simulink model "sim_pla"  (Simulink 2.20)
settings: Solver=FixedStepDiscrete  StartTime=0.0  StopTime=200  MaxStep=.1  RelTol=1e-5  AbsTol=1e-5
values from neighbouring files (symbols this model uses):
  Btot_p = [1.01219559056 -0.470264843111 0.0164957191282 0.00637641130362 -0.0114044125868 0.0367191858533 0.00475496453764 0.0142682114975 -0.02612243686 0.00492786107634 -0.0232059691443 0.00221978390651 ... (36 elements, 6x6)]    [Plant_da.mat]
  Btot_s = [-1.01626574689 2.87547182252 0.160783159509 -0.0616056082235 0.415835595232 -0.0519110171366 -0.981144722525 0.331237826324 0.0458866161445 0.0273695758621 -0.450541570766 0.161910461736 ... (36 elements, 6x6)]    [Plant_da.mat]
  Dtot_p = [0.513358369793  0.0351099859011  0.00780615785705; 0.00923678162985  0.40412781442  0.00373697732041; 0.000710321631108  0.27377444097  0.302765835746]    [Plant_da.mat]
  Dtot_s = [1.88799295885 1.15607702775 1.0967215675 -0.0862589557053 -0.000817934293654 -0.111851597277 2.17273827487 1.17822487272 1.10291377498 0.0376770859254 -0.0289504261378 0.0426395979727 ... (18 elements, 3x6)]    [Plant_da.mat]
  Ftot_p = [-10 5 0 0 0 0 -5 2.40692882292e-15 0 0 0 0 ... (36 elements, 6x6)]    [Plant_da.mat]
  Ftot_s = [-20 10 0 0 0 0 -10 5.05150120952e-15 0 0 0 0 ... (36 elements, 6x6)]    [Plant_da.mat]
  knot_a3_p = [200 1400]    [Plant_da.mat]
  knot_a3_s = [200 1400]    [Plant_da.mat]
  knot_a5_p = [200 1400]    [Plant_da.mat]
  knot_a5_s = [0 1]    [Plant_da.mat]
  knot_d_p = [200 1400]    [Plant_da.mat]
  knot_d_s = [0 1]    [Plant_da.mat]
  knot_u_p = [200 1400]    [Plant_da.mat]
  knot_u_s = [0 1]    [Plant_da.mat]
  knot_y_p = [200 1400]    [Plant_da.mat]
  knot_y_s = [200 1400]    [Plant_da.mat]
  Ltot_p = [-1.64126952333 0.984947018254 0 0 0 0 -0.233477858246 0.0041951537679 0 0 0 0 ... (54 elements, 6x9)]    [Plant_da.mat]
  Ltot_s = [-2.86862859726 1.57424910459 0 0 0 0 -0.0579168602778 -0.011710441158 0 0 0 0 ... (72 elements, 6x12)]    [Plant_da.mat]
  M3_p = [-0.061197222075 8.55026347734 0 0 0 0 7.49858890056 23.7640569756 0 0 0 0 ... (72 elements, 6x12)]    [Plant_da.mat]
  M3_s = [-0.00930250944473 1.93496177148 0 0 0 0 -0.0214766871049 10.7782036277 0 0 0 0 ... (36 elements, 6x6)]    [Plant_da.mat]
  M5_p = [9.76740961374 0 0 -13.0234685756 0 0 -3.35875871132 0 0 0 -0.663402612193 0 ... (27 elements, 3x9)]    [Plant_da.mat]
  M5_s = [-3.17982066424  0  0; 0  -1.6903608647  0; 0  0  -1.55540118092]    [Plant_da.mat]
  ninp_p = 3    [Plant_da.mat]
  ninp_s = 3    [Plant_da.mat]
  noutp_p = 3    [Plant_da.mat]
  noutp_s = 3    [Plant_da.mat]
  order_a3_p = [0 1 2 3]    [Plant_da.mat]
  order_a3_s = [0 1]    [Plant_da.mat]
  order_a5_p = [0 1 2]    [Plant_da.mat]
  order_a5_s = 1    [Plant_da.mat]
  order_d_p = 0    [Plant_da.mat]
  order_d_s = [0 1]    [Plant_da.mat]
  order_u_p = [0 3]    [Plant_da.mat]
  order_u_s = [0 1]    [Plant_da.mat]
  order_y_p = [0 1 3]    [Plant_da.mat]
  order_y_s = [0 1 2 3]    [Plant_da.mat]
  TSAMPLEP = 0.00833333333333    [Plant_da.mat]
  xx0_p = [-43.6952648027 46.4302892278 -75.6051233614 37.0208850933 -65.9903404423 60.1627507041]    [Plant_da.mat]
  xx0_s = [-76.0618282874 11.7629910946 -77.2669838113 13.8232604668 -77.7589073013 10.6536765168]    [Plant_da.mat]
undefined symbols (not defined in the file or in its folder): legev_bv
settings Model: SaveTime=off  SaveOutput=off  ConsistencyChecking=off  RTWPlaceOutputsASAP=off

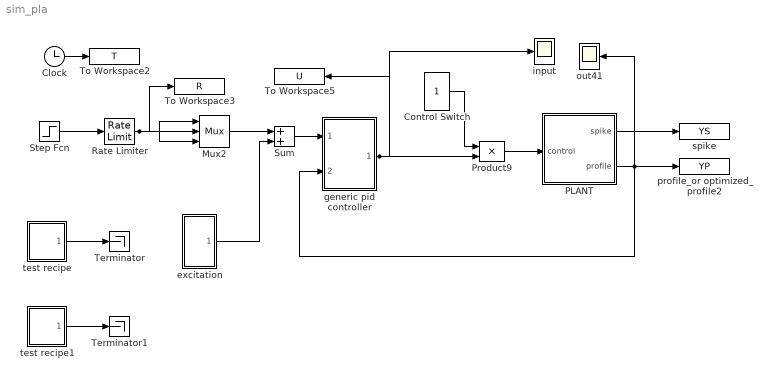
== system sim_pla ==
  Clock : Clock
  Control Switch : Constant  Value=1
  Mux2 : Mux  Inputs=3
  PLANT : Subsystem
      mask init:
      | load 'plant_da'
  Product9 : Product  Inputs=2
  Rate Limiter : RateLimiter  RisingSlewLimit=15  FallingSlewLimit=-5
  Step Fcn : Step  Time=30  Before=550  After=800
  Sum : Sum  Inputs=++
  Terminator : Terminator
  Terminator1 : Terminator
  To Workspace2 : ToWorkspace  VariableName=T  SampleTime=0
      settings: Buffer=25000
  To Workspace3 : ToWorkspace  VariableName=R  SampleTime=0
      settings: Buffer=25000
  To Workspace5 : ToWorkspace  VariableName=U  SampleTime=0
      settings: Buffer=25000
  excitation : Subsystem
      mask init:
      | load 'excit'
  generic pid controller : Subsystem
  input : Scope
      settings: TickLabels=on  TimeRange=200  YMin=0  YMax=1  SaveToWorkspace=off  SaveName=ScopeData  MaxRows=25000  SampleInput=on
  out41 : Scope
      settings: TickLabels=on  TimeRange=200  YMin=500  YMax=1000  SaveToWorkspace=off  SaveName=ScopeData  MaxRows=25000  SampleInput=on
  profile_or optimized_profile2 : ToWorkspace  VariableName=YP  SampleTime=0
      settings: Buffer=25000
  spike : ToWorkspace  VariableName=YS  SampleTime=0
      settings: Buffer=25000
  test recipe : Subsystem  mask(Repeating table){@1=[0     20    35  95  96  200], @2=[550 550 800 800 600 600]}
      mask prompts: @1 "Time values:"; @2 "Output values:"
      mask help:
      | Repeating table.
      | Enter values of time and output for first cycle.
      mask init:
      | period = max(@1); t = @1; y = @2;
      mask Help: Repeats cycle given in table. Time values should be monotonically increasing.
      mask Display: plot([t,t+period,t+2*period],[y,y,y])
  test recipe1 : Subsystem  mask(Repeating table){@1=[0     20    21  95  96  200], @2=[550 550 800 800 600 600]}
      mask prompts: @1 "Time values:"; @2 "Output values:"
      mask help:
      | Repeating table.
      | Enter values of time and output for first cycle.
      mask init:
      | period = max(@1); t = @1; y = @2;
      mask Help: Repeats cycle given in table. Time values should be monotonically increasing.
      mask Display: plot([t,t+period,t+2*period],[y,y,y])
  wires:
  Clock/1 -> To Workspace2/1
  Control Switch/1 -> Product9/1
  Product9/1 -> PLANT/1(control)
  Rate Limiter/1 -> To Workspace3/1, Mux2/1, Mux2/2, Mux2/3
  generic pid controller/1(out_1) -> Product9/2, To Workspace5/1, input/1
  Mux2/1 -> Sum/1
  Sum/1 -> generic pid controller/1(reference)
  PLANT/2(profile) -> generic pid controller/2(output), profile_or optimized_profile2/1, out41/1
  PLANT/1(spike) -> spike/1
  excitation/1(Out1) -> Sum/2
  test recipe/1(out_1) -> Terminator/1
  Step Fcn/1 -> Rate Limiter/1
  test recipe1/1(out_1) -> Terminator1/1

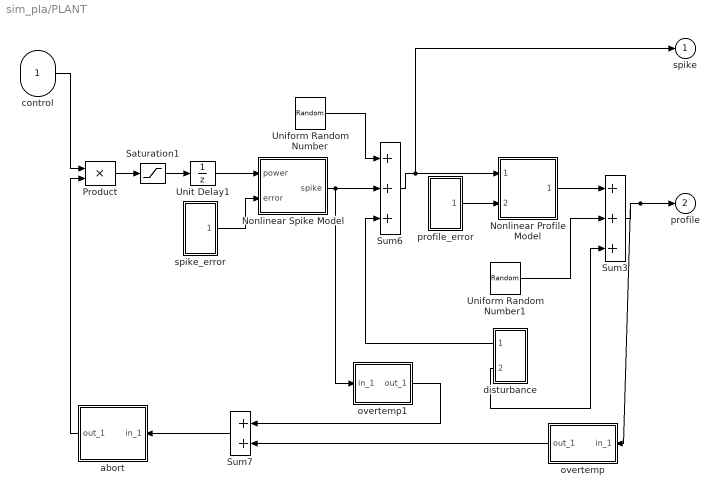
== system sim_pla/PLANT ==
  control : Inport  Port=1  PortWidth=-1  SampleTime=-1
  Nonlinear Profile Model : Subsystem
  Nonlinear Spike Model : Subsystem
  Product : Product  Inputs=2
  Saturation1 : Saturate  UpperLimit=[1 1 1]  LowerLimit=[0 0 0]
  Sum3 : Sum  Inputs=+++
  Sum6 : Sum  Inputs=+++
  Sum7 : Sum  Orientation=left  Inputs=++
  Uniform Random Number : UniformRandomNumber  Minimum=-.2  Maximum=.2  Seed=0  SampleTime=.5/60
  Uniform Random Number1 : UniformRandomNumber  Minimum=-.1  Maximum=.1  Seed=0  SampleTime=.5/60
  Unit Delay1 : UnitDelay  X0=0  SampleTime=TSAMPLEP
  abort : Subsystem  Orientation=left
  disturbance : Subsystem  Orientation=left
  overtemp : Subsystem  Orientation=left
  overtemp1 : Subsystem
  profile_error : Subsystem
  spike_error : Subsystem
  spike : Outport  Port=1  InitialOutput=0
  profile : Outport  Port=2  InitialOutput=0
  wires:
  Nonlinear Profile Model/1(profile) -> Sum3/1
  Uniform Random Number/1 -> Sum6/1
  Product/1 -> Saturation1/1
  Saturation1/1 -> Unit Delay1/1
  Unit Delay1/1 -> Nonlinear Spike Model/1(power)
  control/1 -> Product/1
  spike_error/1(out_1) -> Nonlinear Spike Model/2(error)
  profile_error/1(out_1) -> Nonlinear Profile Model/2(error)
  Uniform Random Number1/1 -> Sum3/2
  Nonlinear Spike Model/1(spike) -> Sum6/2, overtemp1/1(in_1)
  Sum3/1 -> profile/1, overtemp/1(in_1)
  Sum6/1 -> Nonlinear Profile Model/1(spike1), spike/1
  abort/1(out_1) -> Product/2
  Sum7/1 -> abort/1(in_1)
  overtemp1/1(out_1) -> Sum7/1
  overtemp/1(out_1) -> Sum7/2
  disturbance/1(spike) -> Sum6/3
  disturbance/2(profile) -> Sum3/3

== system sim_pla/excitation ==
  From  Workspace : FromWorkspace  VariableName=[TX,RX]
  Gain : Gain  Gain=1
  Out1 : Outport  Port=1  InitialOutput=0
  wires:
  Gain/1 -> Out1/1
  From  Workspace/1 -> Gain/1

== system sim_pla/generic pid controller ==
  note: 2.9873e-002  2.3770e+000  1.1004e+000
      |   5.8485e-002  3.6863e+000  1.3216e+000
      |   3.1318e-002  1.7040e+000  2.9610e+000
  reference : Inport  Port=1  PortWidth=-1  SampleTime=-1
  output : Inport  Port=2  PortWidth=-1  SampleTime=-1
  "AW-PID " : Subsystem  mask(Anti-windup PID ){SAM=.1, TF=0.1, DT=.5/60}
      mask prompts: SAM "Gain kp - Integral time ki - Derivative time kd"; TF "Pseudo-derivative filter time constant"; DT "Error lowpass filter Time constant"
      mask help: Discrete PID with Anti-windup and with lowpass filter
      mask init:
      | kp=@1(1);ki=@1(2);kd=@1(3);umax=@5(1);umin=@5(2);
      mask Display: disp('AW-PID+filter')
  AW-PID 1 : Subsystem  mask(Anti-windup PID ){@1=[.047, 1.96, 1.2], @2=.1, @3=0.1, @4=.5/60, @5=[1 0]}
      mask prompts: @1 "Gain kp - Integral time ki - Derivative time kd"; @2 "Pseudo-derivative filter time constant"; @3 "Error lowpass filter Time constant"; @4 "Sampling Time"; @5 "Saturation Limits [umax umin]"
      mask help: Discrete PID with Anti-windup and with lowpass filter
      mask init:
      | kp=@1(1);ki=@1(2);kd=@1(3);SAM=@2;TF=@3;DT=@4;umax=@5(1);umin=@5(2);
      mask Display: disp('AW-PID+filter')
  AW-PID 2 : Subsystem  mask(Anti-windup PID ){@1=[.027, 1.66, 1.9], @2=.1, @3=0.1, @4=.5/60, @5=[1 0]}
      mask prompts: @1 "Gain kp - Integral time ki - Derivative time kd"; @2 "Pseudo-derivative filter time constant"; @3 "Error lowpass filter Time constant"; @4 "Sampling Time"; @5 "Saturation Limits [umax umin]"
      mask help: Discrete PID with Anti-windup and with lowpass filter
      mask init:
      | kp=@1(1);ki=@1(2);kd=@1(3);SAM=@2;TF=@3;DT=@4;umax=@5(1);umin=@5(2);
      mask Display: disp('AW-PID+filter')
  Demux : Demux  Outputs=3
  Demux1 : Demux  Outputs=3
  Mux2 : Mux  Inputs=3
  out_1 : Outport  Port=1  InitialOutput=0
  wires:
  AW-PID 2/1(Input to system) -> Mux2/3
  "AW-PID "/1(Input to system) -> Mux2/1
  AW-PID 1/1(Input to system) -> Mux2/2
  Mux2/1 -> out_1/1
  reference/1 -> Demux/1
  Demux/1 -> "AW-PID "/1(Set point)
  Demux/2 -> AW-PID 1/1(Set point)
  Demux/3 -> AW-PID 2/1(Set point)
  Demux1/3 -> AW-PID 2/2(System Output)
  output/1 -> Demux1/1
  Demux1/2 -> AW-PID 1/2(System Output)
  Demux1/1 -> "AW-PID "/2(System Output)

== system sim_pla/test recipe ==
  Clock : Clock
  Fcn1 : Fcn  Expr=rem(u[1],period)
  Look-Up Table : Lookup  InputValues=t  OutputValues=y
  out_1 : Outport  Port=1  InitialOutput=0
  wires:
  Look-Up Table/1 -> out_1/1
  Clock/1 -> Fcn1/1
  Fcn1/1 -> Look-Up Table/1

== system sim_pla/test recipe1 ==
  Clock : Clock
  Fcn1 : Fcn  Expr=rem(u[1],period)
  Look-Up Table : Lookup  InputValues=t  OutputValues=y
  out_1 : Outport  Port=1  InitialOutput=0
  wires:
  Look-Up Table/1 -> out_1/1
  Clock/1 -> Fcn1/1
  Fcn1/1 -> Look-Up Table/1

== system sim_pla/PLANT/Nonlinear Profile Model ==
  spike1 : Inport  Port=1  PortWidth=-1  SampleTime=-1
  error : Inport  Port=2  PortWidth=-1  SampleTime=-1
  Denominator Block : Subsystem  Orientation=left
  Numerator Block : Subsystem
  Sum : Sum  Inputs=+++
  profile : Outport  Port=1  InitialOutput=0
  wires:
  Sum/1 -> profile/1, Denominator Block/1(in_1)
  Numerator Block/1(out_1) -> Sum/1
  spike1/1 -> Numerator Block/1(in_1)
  Denominator Block/1(out_1) -> Sum/3
  error/1 -> Sum/2

== system sim_pla/PLANT/Nonlinear Spike Model ==
  power : Inport  Port=1  PortWidth=-1  SampleTime=-1
  error : Inport  Port=2  PortWidth=-1  SampleTime=-1
  Denominator Block : Subsystem  Orientation=left
  Numerator Block : Subsystem
  Sum : Sum  Inputs=+++
  spike : Outport  Port=1  InitialOutput=0
  wires:
  power/1 -> Numerator Block/1(in_1)
  Numerator Block/1(out_1) -> Sum/1
  Sum/1 -> spike/1, Denominator Block/1(in_1)
  Denominator Block/1(out_1) -> Sum/3
  error/1 -> Sum/2

== system sim_pla/PLANT/abort ==
  in_1 : Inport  Port=1  PortWidth=-1  SampleTime=-1
  Abs : Abs
  Constant : Constant  Value=1
  Relational Operator : RelationalOperator  Operator=>=
  Sum : Sum  Inputs=++
  Sum1 : Sum  Inputs=-+
  Unit Delay3 : UnitDelay  X0=0  SampleTime=TSAMPLEP
  out_1 : Outport  Port=1  InitialOutput=0
  wires:
  Sum1/1 -> out_1/1
  Relational Operator/1 -> Sum1/1
  Constant/1 -> Sum1/2, Relational Operator/2
  Unit Delay3/1 -> Relational Operator/1, Sum/2
  in_1/1 -> Abs/1
  Sum/1 -> Unit Delay3/1
  Abs/1 -> Sum/1

== system sim_pla/PLANT/disturbance ==
  Discrete Transfer Fcn : DiscreteTransferFcn  Orientation=left  Numerator=[1]  Denominator=[.5/TSAMPLEP 1-.5/TSAMPLEP]  SampleTime=TSAMPLEP
  Discrete Transfer Fcn1 : DiscreteTransferFcn  Orientation=left  Numerator=[10/TSAMPLEP -10/TSAMPLEP]  Denominator=[10/TSAMPLEP 1-10/TSAMPLEP]  SampleTime=TSAMPLEP
  Discrete Transfer Fcn2 : DiscreteTransferFcn  Orientation=left  Numerator=[1]  Denominator=[2/TSAMPLEP 1-2/TSAMPLEP]  SampleTime=TSAMPLEP
  Sum4 : Sum  Orientation=left  Inputs=++
  disturbance : Step  Orientation=left  Time=55  Before=0  After=10
  disturbance2 : Step  Orientation=left  Time=75  Before=0  After=-5
  spike : Outport  Orientation=left  Port=1  InitialOutput=0
  profile : Outport  Orientation=left  Port=2  InitialOutput=0
  wires:
  Discrete Transfer Fcn1/1 -> profile/1
  Discrete Transfer Fcn/1 -> spike/1
  Sum4/1 -> Discrete Transfer Fcn/1, Discrete Transfer Fcn1/1
  disturbance/1 -> Sum4/1
  disturbance2/1 -> Discrete Transfer Fcn2/1
  Discrete Transfer Fcn2/1 -> Sum4/2

== system sim_pla/PLANT/overtemp ==
  in_1 : Inport  Port=1  PortWidth=-1  SampleTime=-1
  Constant : Constant  Value=950
  Relational Operator : RelationalOperator  Operator=>
  out_1 : Outport  Port=1  InitialOutput=0
  wires:
  in_1/1 -> Relational Operator/1
  Relational Operator/1 -> out_1/1
  Constant/1 -> Relational Operator/2

== system sim_pla/PLANT/overtemp1 ==
  in_1 : Inport  Port=1  PortWidth=-1  SampleTime=-1
  Constant : Constant  Value=1000
  Relational Operator : RelationalOperator  Operator=>
  out_1 : Outport  Port=1  InitialOutput=0
  wires:
  in_1/1 -> Relational Operator/1
  Relational Operator/1 -> out_1/1
  Constant/1 -> Relational Operator/2

== system sim_pla/PLANT/profile_error ==
  Mux1 : Mux  Inputs=3
  prof error : Subsystem  mask(Repeating table){@1=TEPRO, @2=FEP1}
      mask prompts: @1 "Time values:"; @2 "Output values:"
      mask help:
      | Repeating table.
      | Enter values of time and output for first cycle.
      mask init:
      | period = max(@1); t = @1; y = @2;
      mask Help: Repeats cycle given in table. Time values should be monotonically increasing.
      mask Display: plot([t,t+period,t+2*period],[y,y,y])
  prof error1 : Subsystem  mask(Repeating table){@1=TEPRO, @2=FEP2}
      mask prompts: @1 "Time values:"; @2 "Output values:"
      mask help:
      | Repeating table.
      | Enter values of time and output for first cycle.
      mask init:
      | period = max(@1); t = @1; y = @2;
      mask Help: Repeats cycle given in table. Time values should be monotonically increasing.
      mask Display: plot([t,t+period,t+2*period],[y,y,y])
  prof error2 : Subsystem  mask(Repeating table){@1=TEPRO, @2=FEP3}
      mask prompts: @1 "Time values:"; @2 "Output values:"
      mask help:
      | Repeating table.
      | Enter values of time and output for first cycle.
      mask init:
      | period = max(@1); t = @1; y = @2;
      mask Help: Repeats cycle given in table. Time values should be monotonically increasing.
      mask Display: plot([t,t+period,t+2*period],[y,y,y])
  out_1 : Outport  Port=1  InitialOutput=0
  wires:
  Mux1/1 -> out_1/1
  prof error/1(out_1) -> Mux1/1
  prof error1/1(out_1) -> Mux1/2
  prof error2/1(out_1) -> Mux1/3

== system sim_pla/PLANT/spike_error ==
  Mux1 : Mux  Inputs=3
  spike error : Subsystem  mask(Repeating table){@1=TEPRO, @2=FES1}
      mask prompts: @1 "Time values:"; @2 "Output values:"
      mask help:
      | Repeating table.
      | Enter values of time and output for first cycle.
      mask init:
      | period = max(@1); t = @1; y = @2;
      mask Help: Repeats cycle given in table. Time values should be monotonically increasing.
      mask Display: plot([t,t+period,t+2*period],[y,y,y])
  spike error1 : Subsystem  mask(Repeating table){@1=TEPRO, @2=FES2}
      mask prompts: @1 "Time values:"; @2 "Output values:"
      mask help:
      | Repeating table.
      | Enter values of time and output for first cycle.
      mask init:
      | period = max(@1); t = @1; y = @2;
      mask Help: Repeats cycle given in table. Time values should be monotonically increasing.
      mask Display: plot([t,t+period,t+2*period],[y,y,y])
  spike error2 : Subsystem  mask(Repeating table){@1=TEPRO, @2=FES3}
      mask prompts: @1 "Time values:"; @2 "Output values:"
      mask help:
      | Repeating table.
      | Enter values of time and output for first cycle.
      mask init:
      | period = max(@1); t = @1; y = @2;
      mask Help: Repeats cycle given in table. Time values should be monotonically increasing.
      mask Display: plot([t,t+period,t+2*period],[y,y,y])
  out_1 : Outport  Port=1  InitialOutput=0
  wires:
  Mux1/1 -> out_1/1
  spike error/1(out_1) -> Mux1/1
  spike error1/1(out_1) -> Mux1/2
  spike error2/1(out_1) -> Mux1/3

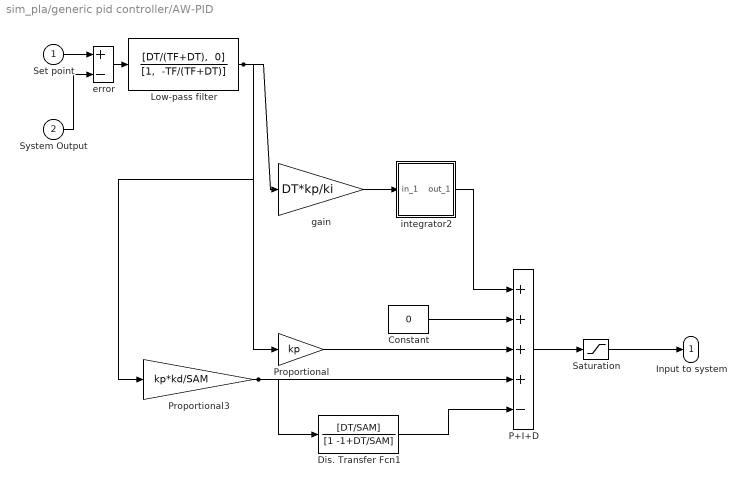
== system sim_pla/generic pid controller/AW-PID  ==
  Set point : Inport  Port=1  PortWidth=-1  SampleTime=-1
  System Output : Inport  Port=2  PortWidth=-1  SampleTime=-1
  Constant : Constant  Value=0
  Dis. Transfer Fcn1 : DiscreteTransferFcn  Numerator=[DT/SAM]  Denominator=[1 -1+DT/SAM]  SampleTime=DT
  Low-pass filter : DiscreteTransferFcn  Numerator="[DT/(TF+DT),  0]"  Denominator="[1,  -TF/(TF+DT)]"  SampleTime=DT
  P+I+D : Sum  Inputs=++++-
  Proportional : Gain  Gain=kp
  Proportional3 : Gain  Gain=kp*kd/SAM
  Saturation : Saturate  UpperLimit=umax  LowerLimit=umin
  error : Sum  Inputs=+-
  gain : Gain  Gain=DT*kp/ki
  integrator2 : Subsystem  mask(Anti windup intgrator){@1=umax, @2=umin, @3=DT}
      mask prompts: @1 "umax"; @2 "umin"; @3 "sampling time"
      mask help: Integral with anti-windup
      mask init:
      | umax=@1 ; umin =@2 ;DT=@3;
      mask Display: disp('DT-I-AW')
  Input to system : Outport  Port=1  InitialOutput=0
  wires:
  integrator2/1(out_1) -> P+I+D/1
  error/1 -> Low-pass filter/1
  Set point/1 -> error/1
  System Output/1 -> error/2
  Low-pass filter/1 -> Proportional/1, Proportional3/1, gain/1
  Dis. Transfer Fcn1/1 -> P+I+D/5
  Proportional3/1 -> Dis. Transfer Fcn1/1, P+I+D/4
  Proportional/1 -> P+I+D/3
  gain/1 -> integrator2/1(in_1)
  P+I+D/1 -> Saturation/1
  Saturation/1 -> Input to system/1
  Constant/1 -> P+I+D/2

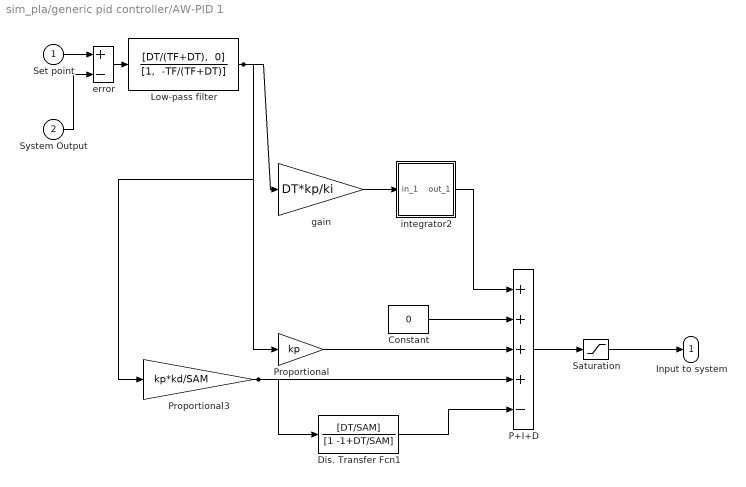
== system sim_pla/generic pid controller/AW-PID 1 ==
  Set point : Inport  Port=1  PortWidth=-1  SampleTime=-1
  System Output : Inport  Port=2  PortWidth=-1  SampleTime=-1
  Constant : Constant  Value=0
  Dis. Transfer Fcn1 : DiscreteTransferFcn  Numerator=[DT/SAM]  Denominator=[1 -1+DT/SAM]  SampleTime=DT
  Low-pass filter : DiscreteTransferFcn  Numerator="[DT/(TF+DT),  0]"  Denominator="[1,  -TF/(TF+DT)]"  SampleTime=DT
  P+I+D : Sum  Inputs=++++-
  Proportional : Gain  Gain=kp
  Proportional3 : Gain  Gain=kp*kd/SAM
  Saturation : Saturate  UpperLimit=umax  LowerLimit=umin
  error : Sum  Inputs=+-
  gain : Gain  Gain=DT*kp/ki
  integrator2 : Subsystem  mask(Anti windup intgrator){@1=umax, @2=umin, @3=DT}
      mask prompts: @1 "umax"; @2 "umin"; @3 "sampling time"
      mask help: Integral with anti-windup
      mask init:
      | umax=@1 ; umin =@2 ;DT=@3;
      mask Display: disp('DT-I-AW')
  Input to system : Outport  Port=1  InitialOutput=0
  wires:
  integrator2/1(out_1) -> P+I+D/1
  error/1 -> Low-pass filter/1
  Set point/1 -> error/1
  System Output/1 -> error/2
  Low-pass filter/1 -> Proportional/1, Proportional3/1, gain/1
  Dis. Transfer Fcn1/1 -> P+I+D/5
  Proportional3/1 -> Dis. Transfer Fcn1/1, P+I+D/4
  Proportional/1 -> P+I+D/3
  gain/1 -> integrator2/1(in_1)
  P+I+D/1 -> Saturation/1
  Saturation/1 -> Input to system/1
  Constant/1 -> P+I+D/2

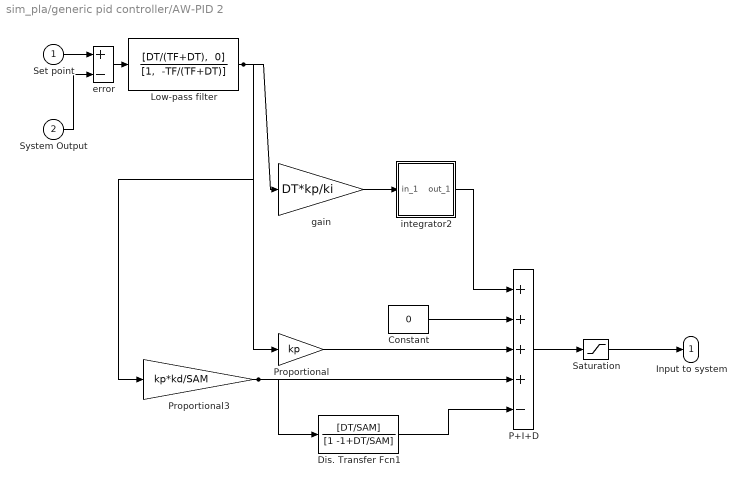
== system sim_pla/generic pid controller/AW-PID 2 ==
  Set point : Inport  Port=1  PortWidth=-1  SampleTime=-1
  System Output : Inport  Port=2  PortWidth=-1  SampleTime=-1
  Constant : Constant  Value=0
  Dis. Transfer Fcn1 : DiscreteTransferFcn  Numerator=[DT/SAM]  Denominator=[1 -1+DT/SAM]  SampleTime=DT
  Low-pass filter : DiscreteTransferFcn  Numerator="[DT/(TF+DT),  0]"  Denominator="[1,  -TF/(TF+DT)]"  SampleTime=DT
  P+I+D : Sum  Inputs=++++-
  Proportional : Gain  Gain=kp
  Proportional3 : Gain  Gain=kp*kd/SAM
  Saturation : Saturate  UpperLimit=umax  LowerLimit=umin
  error : Sum  Inputs=+-
  gain : Gain  Gain=DT*kp/ki
  integrator2 : Subsystem  mask(Anti windup intgrator){@1=umax, @2=umin, @3=DT}
      mask prompts: @1 "umax"; @2 "umin"; @3 "sampling time"
      mask help: Integral with anti-windup
      mask init:
      | umax=@1 ; umin =@2 ;DT=@3;
      mask Display: disp('DT-I-AW')
  Input to system : Outport  Port=1  InitialOutput=0
  wires:
  integrator2/1(out_1) -> P+I+D/1
  error/1 -> Low-pass filter/1
  Set point/1 -> error/1
  System Output/1 -> error/2
  Low-pass filter/1 -> Proportional/1, Proportional3/1, gain/1
  Dis. Transfer Fcn1/1 -> P+I+D/5
  Proportional3/1 -> Dis. Transfer Fcn1/1, P+I+D/4
  Proportional/1 -> P+I+D/3
  gain/1 -> integrator2/1(in_1)
  P+I+D/1 -> Saturation/1
  Saturation/1 -> Input to system/1
  Constant/1 -> P+I+D/2

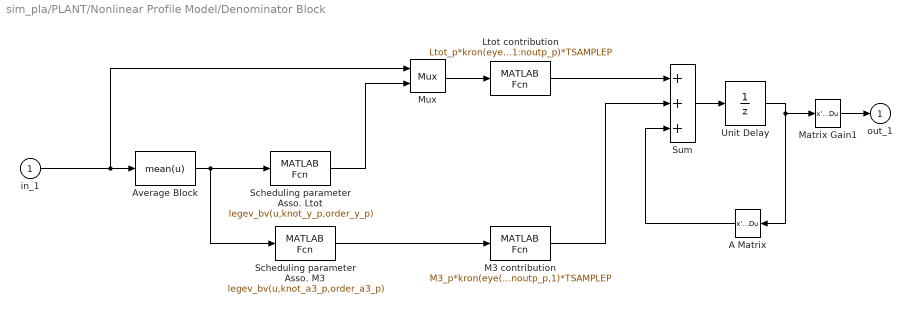
== system sim_pla/PLANT/Nonlinear Profile Model/Denominator Block ==
  in_1 : Inport  Port=1  PortWidth=-1  SampleTime=-1
  A Matrix : StateSpace  Orientation=left  A=[]  B=[]  C=[]  D=K  X0=0  mask(Matrix Gain){@1=(eye(size(Ftot_p))+TSAMPLEP*Ftot_p)}
      mask prompts: @1 "Gain matrix:"
      mask help: Matrix Gain.
      mask init:
      | K = @1;
      mask Help: Multiplies input vector by entered matrix to produce output vector (y=Au).
      mask Display: disp('K')
  Average Block : MATLABFcn  MATLABFcn=mean(u)  OutputWidth=1
  Ltot contribution : MATLABFcn  MATLABFcn=Ltot_p*kron(eye(noutp_p),u(noutp_p+1:noutp_p+length(order_y_p)))*u(1:noutp_p)*TSAMPLEP  OutputWidth=length(Ftot_p)
  M3 contribution : MATLABFcn  MATLABFcn=M3_p*kron(eye(noutp_p),u)*ones(noutp_p,1)*TSAMPLEP  OutputWidth=length(Ftot_p)
  Matrix Gain1 : StateSpace  A=[]  B=[]  C=[]  D=K  X0=0  mask(Matrix Gain){@1=Qtot_p}
      mask prompts: @1 "Gain matrix:"
      mask help: Matrix Gain.
      mask init:
      | K = @1;
      mask Help: Multiplies input vector by entered matrix to produce output vector (y=Au).
      mask Display: disp('K')
  Mux : Mux  Inputs=2
  Scheduling parameter Asso. Ltot : MATLABFcn  MATLABFcn=legev_bv(u,knot_y_p,order_y_p)  OutputWidth=length(order_y_p)
  Scheduling parameter Asso. M3 : MATLABFcn  MATLABFcn=legev_bv(u,knot_a3_p,order_a3_p)  OutputWidth=length(order_a3_p)
  Sum : Sum  Inputs=+++
  Unit Delay : UnitDelay  X0=0  SampleTime=TSAMPLEP
  out_1 : Outport  Port=1  InitialOutput=0
  wires:
  in_1/1 -> Average Block/1, Mux/1
  Average Block/1 -> Scheduling parameter Asso. Ltot/1, Scheduling parameter Asso. M3/1
  Unit Delay/1 -> A Matrix/1, Matrix Gain1/1
  A Matrix/1 -> Sum/3
  Scheduling parameter Asso. M3/1 -> M3 contribution/1
  M3 contribution/1 -> Sum/2
  Ltot contribution/1 -> Sum/1
  Scheduling parameter Asso. Ltot/1 -> Mux/2
  Mux/1 -> Ltot contribution/1
  Sum/1 -> Unit Delay/1
  Matrix Gain1/1 -> out_1/1

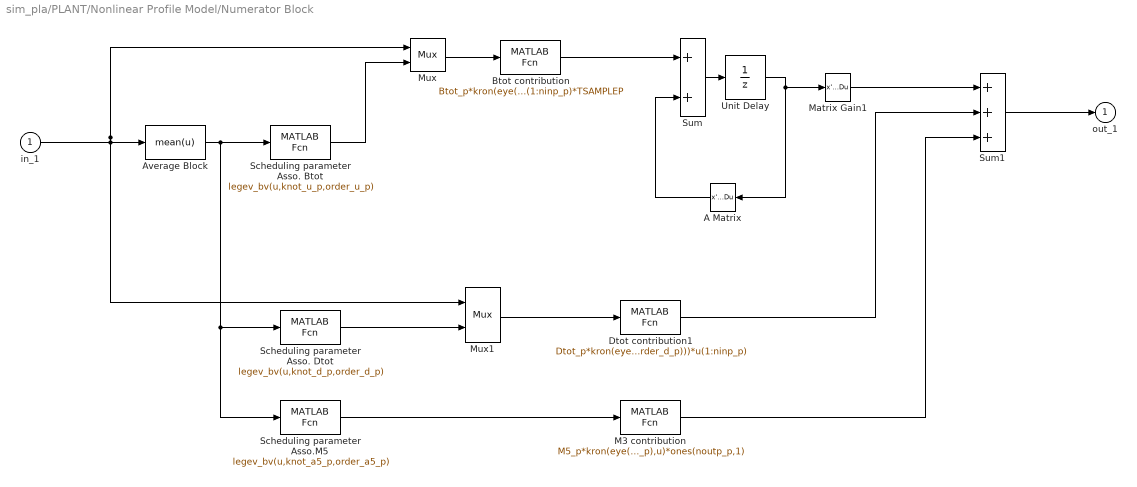
== system sim_pla/PLANT/Nonlinear Profile Model/Numerator Block ==
  in_1 : Inport  Port=1  PortWidth=-1  SampleTime=-1
  A Matrix : StateSpace  Orientation=left  A=[]  B=[]  C=[]  D=K  X0=0  mask(Matrix Gain){@1=(eye(size(Ftot_p))+TSAMPLEP*Ftot_p)}
      mask prompts: @1 "Gain matrix:"
      mask help: Matrix Gain.
      mask init:
      | K = @1;
      mask Help: Multiplies input vector by entered matrix to produce output vector (y=Au).
      mask Display: disp('K')
  Average Block : MATLABFcn  MATLABFcn=mean(u)  OutputWidth=1
  Btot contribution : MATLABFcn  MATLABFcn=Btot_p*kron(eye(noutp_p),u(ninp_p+1:ninp_p+length(order_u_p)))*u(1:ninp_p)*TSAMPLEP  OutputWidth=length(Ftot_p)
  Dtot contribution1 : MATLABFcn  MATLABFcn=Dtot_p*kron(eye(noutp_p),u(ninp_p+1:ninp_p+length(order_d_p)))*u(1:ninp_p)  OutputWidth=noutp_p
  M3 contribution : MATLABFcn  MATLABFcn=M5_p*kron(eye(noutp_p),u)*ones(noutp_p,1)  OutputWidth=noutp_p
  Matrix Gain1 : StateSpace  A=[]  B=[]  C=[]  D=K  X0=0  mask(Matrix Gain){@1=Qtot_p}
      mask prompts: @1 "Gain matrix:"
      mask help: Matrix Gain.
      mask init:
      | K = @1;
      mask Help: Multiplies input vector by entered matrix to produce output vector (y=Au).
      mask Display: disp('K')
  Mux : Mux  Inputs=2
  Mux1 : Mux  Inputs=2
  Scheduling parameter Asso. Btot : MATLABFcn  MATLABFcn=legev_bv(u,knot_u_p,order_u_p)  OutputWidth=length(order_u_p)
  Scheduling parameter Asso. Dtot : MATLABFcn  MATLABFcn=legev_bv(u,knot_d_p,order_d_p)  OutputWidth=length(order_d_p)
  Scheduling parameter Asso.M5 : MATLABFcn  MATLABFcn=legev_bv(u,knot_a5_p,order_a5_p)  OutputWidth=length(order_a5_p)
  Sum : Sum  Inputs=++
  Sum1 : Sum  Inputs=+++
  Unit Delay : UnitDelay  X0=xx0_p(:,1)  SampleTime=TSAMPLEP
  out_1 : Outport  Port=1  InitialOutput=0
  wires:
  Sum/1 -> Unit Delay/1
  Mux/1 -> Btot contribution/1
  Scheduling parameter Asso. Btot/1 -> Mux/2
  Btot contribution/1 -> Sum/1
  Unit Delay/1 -> A Matrix/1, Matrix Gain1/1
  A Matrix/1 -> Sum/2
  in_1/1 -> Average Block/1, Mux/1, Mux1/1
  Scheduling parameter Asso. Dtot/1 -> Mux1/2
  Mux1/1 -> Dtot contribution1/1
  Average Block/1 -> Scheduling parameter Asso. Btot/1, Scheduling parameter Asso. Dtot/1, Scheduling parameter Asso.M5/1
  Scheduling parameter Asso.M5/1 -> M3 contribution/1
  Matrix Gain1/1 -> Sum1/1
  Dtot contribution1/1 -> Sum1/2
  M3 contribution/1 -> Sum1/3
  Sum1/1 -> out_1/1

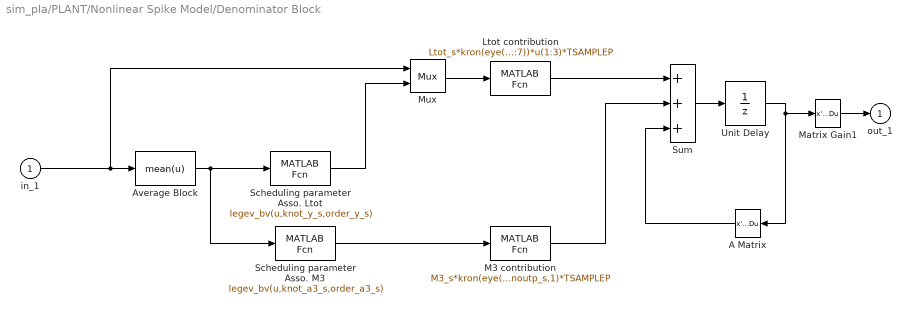
== system sim_pla/PLANT/Nonlinear Spike Model/Denominator Block ==
  in_1 : Inport  Port=1  PortWidth=-1  SampleTime=-1
  A Matrix : StateSpace  Orientation=left  A=[]  B=[]  C=[]  D=K  X0=0  mask(Matrix Gain){@1=(eye(size(Ftot_s))+TSAMPLEP*Ftot_s)}
      mask prompts: @1 "Gain matrix:"
      mask help: Matrix Gain.
      mask init:
      | K = @1;
      mask Help: Multiplies input vector by entered matrix to produce output vector (y=Au).
      mask Display: disp('K')
  Average Block : MATLABFcn  MATLABFcn=mean(u)  OutputWidth=1
  Ltot contribution : MATLABFcn  MATLABFcn=Ltot_s*kron(eye(noutp_s),u(4:7))*u(1:3)*TSAMPLEP  OutputWidth=length(Ftot_s)
  M3 contribution : MATLABFcn  MATLABFcn=M3_s*kron(eye(noutp_s),u)*ones(noutp_s,1)*TSAMPLEP  OutputWidth=length(Ftot_s)
  Matrix Gain1 : StateSpace  A=[]  B=[]  C=[]  D=K  X0=0  mask(Matrix Gain){@1=Qtot_s}
      mask prompts: @1 "Gain matrix:"
      mask help: Matrix Gain.
      mask init:
      | K = @1;
      mask Help: Multiplies input vector by entered matrix to produce output vector (y=Au).
      mask Display: disp('K')
  Mux : Mux  Inputs=2
  Scheduling parameter Asso. Ltot : MATLABFcn  MATLABFcn=legev_bv(u,knot_y_s,order_y_s)  OutputWidth=length(order_y_s)
  Scheduling parameter Asso. M3 : MATLABFcn  MATLABFcn=legev_bv(u,knot_a3_s,order_a3_s)  OutputWidth=length(order_a3_s)
  Sum : Sum  Inputs=+++
  Unit Delay : UnitDelay  X0=0  SampleTime=TSAMPLEP
  out_1 : Outport  Port=1  InitialOutput=0
  wires:
  Matrix Gain1/1 -> out_1/1
  Sum/1 -> Unit Delay/1
  Mux/1 -> Ltot contribution/1
  Scheduling parameter Asso. Ltot/1 -> Mux/2
  Ltot contribution/1 -> Sum/1
  M3 contribution/1 -> Sum/2
  Scheduling parameter Asso. M3/1 -> M3 contribution/1
  A Matrix/1 -> Sum/3
  Unit Delay/1 -> A Matrix/1, Matrix Gain1/1
  Average Block/1 -> Scheduling parameter Asso. Ltot/1, Scheduling parameter Asso. M3/1
  in_1/1 -> Average Block/1, Mux/1

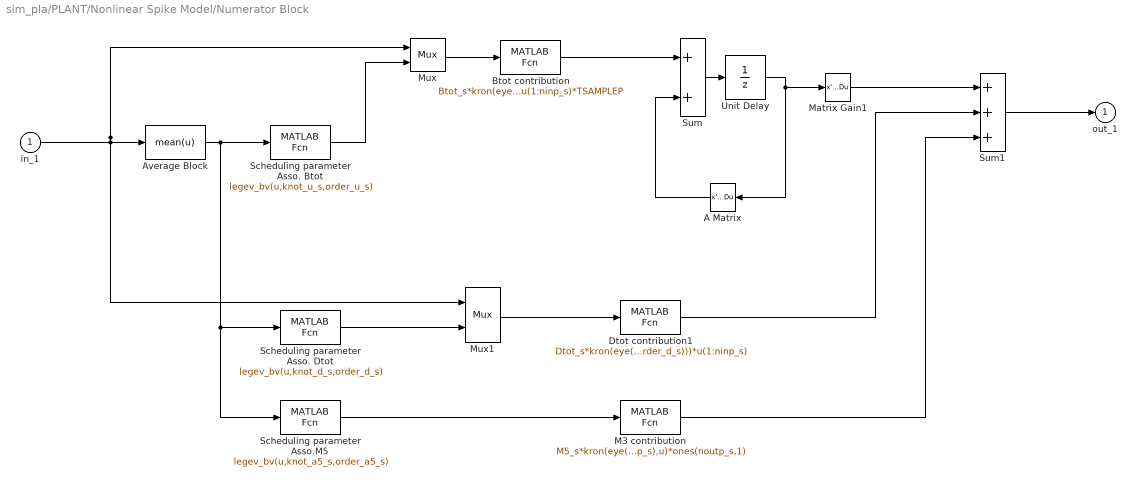
== system sim_pla/PLANT/Nonlinear Spike Model/Numerator Block ==
  in_1 : Inport  Port=1  PortWidth=-1  SampleTime=-1
  A Matrix : StateSpace  Orientation=left  A=[]  B=[]  C=[]  D=K  X0=0  mask(Matrix Gain){@1=(eye(size(Ftot_s))+TSAMPLEP*Ftot_s)}
      mask prompts: @1 "Gain matrix:"
      mask help: Matrix Gain.
      mask init:
      | K = @1;
      mask Help: Multiplies input vector by entered matrix to produce output vector (y=Au).
      mask Display: disp('K')
  Average Block : MATLABFcn  MATLABFcn=mean(u)  OutputWidth=1
  Btot contribution : MATLABFcn  MATLABFcn=Btot_s*kron(eye(noutp_s),u(ninp_s+1:ninp_s+length(order_u_s)))*u(1:ninp_s)*TSAMPLEP  OutputWidth=length(Ftot_s)
  Dtot contribution1 : MATLABFcn  MATLABFcn=Dtot_s*kron(eye(noutp_s),u(ninp_s+1:ninp_s+length(order_d_s)))*u(1:ninp_s)  OutputWidth=noutp_s
  M3 contribution : MATLABFcn  MATLABFcn=M5_s*kron(eye(noutp_s),u)*ones(noutp_s,1)  OutputWidth=noutp_s
  Matrix Gain1 : StateSpace  A=[]  B=[]  C=[]  D=K  X0=0  mask(Matrix Gain){@1=Qtot_s}
      mask prompts: @1 "Gain matrix:"
      mask help: Matrix Gain.
      mask init:
      | K = @1;
      mask Help: Multiplies input vector by entered matrix to produce output vector (y=Au).
      mask Display: disp('K')
  Mux : Mux  Inputs=2
  Mux1 : Mux  Inputs=2
  Scheduling parameter Asso. Btot : MATLABFcn  MATLABFcn=legev_bv(u,knot_u_s,order_u_s)  OutputWidth=length(order_u_s)
  Scheduling parameter Asso. Dtot : MATLABFcn  MATLABFcn=legev_bv(u,knot_d_s,order_d_s)  OutputWidth=length(order_d_s)
  Scheduling parameter Asso.M5 : MATLABFcn  MATLABFcn=legev_bv(u,knot_a5_s,order_a5_s)  OutputWidth=length(order_a5_s)
  Sum : Sum  Inputs=++
  Sum1 : Sum  Inputs=+++
  Unit Delay : UnitDelay  X0=xx0_s(:,1)  SampleTime=TSAMPLEP
  out_1 : Outport  Port=1  InitialOutput=0
  wires:
  Sum1/1 -> out_1/1
  M3 contribution/1 -> Sum1/3
  Dtot contribution1/1 -> Sum1/2
  Matrix Gain1/1 -> Sum1/1
  Scheduling parameter Asso.M5/1 -> M3 contribution/1
  Average Block/1 -> Scheduling parameter Asso. Btot/1, Scheduling parameter Asso. Dtot/1, Scheduling parameter Asso.M5/1
  Mux1/1 -> Dtot contribution1/1
  Scheduling parameter Asso. Dtot/1 -> Mux1/2
  in_1/1 -> Average Block/1, Mux/1, Mux1/1
  A Matrix/1 -> Sum/2
  Unit Delay/1 -> A Matrix/1, Matrix Gain1/1
  Btot contribution/1 -> Sum/1
  Scheduling parameter Asso. Btot/1 -> Mux/2
  Mux/1 -> Btot contribution/1
  Sum/1 -> Unit Delay/1

== system sim_pla/PLANT/profile_error/prof error ==
  Clock : Clock
  Fcn1 : Fcn  Expr=rem(u[1],period)
  Look-Up Table : Lookup  InputValues=t  OutputValues=y
  out_1 : Outport  Port=1  InitialOutput=0
  wires:
  Look-Up Table/1 -> out_1/1
  Clock/1 -> Fcn1/1
  Fcn1/1 -> Look-Up Table/1

== system sim_pla/PLANT/profile_error/prof error1 ==
  Clock : Clock
  Fcn1 : Fcn  Expr=rem(u[1],period)
  Look-Up Table : Lookup  InputValues=t  OutputValues=y
  out_1 : Outport  Port=1  InitialOutput=0
  wires:
  Look-Up Table/1 -> out_1/1
  Clock/1 -> Fcn1/1
  Fcn1/1 -> Look-Up Table/1

== system sim_pla/PLANT/profile_error/prof error2 ==
  Clock : Clock
  Fcn1 : Fcn  Expr=rem(u[1],period)
  Look-Up Table : Lookup  InputValues=t  OutputValues=y
  out_1 : Outport  Port=1  InitialOutput=0
  wires:
  Look-Up Table/1 -> out_1/1
  Clock/1 -> Fcn1/1
  Fcn1/1 -> Look-Up Table/1

== system sim_pla/PLANT/spike_error/spike error ==
  Clock : Clock
  Fcn1 : Fcn  Expr=rem(u[1],period)
  Look-Up Table : Lookup  InputValues=t  OutputValues=y
  out_1 : Outport  Port=1  InitialOutput=0
  wires:
  Look-Up Table/1 -> out_1/1
  Clock/1 -> Fcn1/1
  Fcn1/1 -> Look-Up Table/1

== system sim_pla/PLANT/spike_error/spike error1 ==
  Clock : Clock
  Fcn1 : Fcn  Expr=rem(u[1],period)
  Look-Up Table : Lookup  InputValues=t  OutputValues=y
  out_1 : Outport  Port=1  InitialOutput=0
  wires:
  Look-Up Table/1 -> out_1/1
  Clock/1 -> Fcn1/1
  Fcn1/1 -> Look-Up Table/1

== system sim_pla/PLANT/spike_error/spike error2 ==
  Clock : Clock
  Fcn1 : Fcn  Expr=rem(u[1],period)
  Look-Up Table : Lookup  InputValues=t  OutputValues=y
  out_1 : Outport  Port=1  InitialOutput=0
  wires:
  Look-Up Table/1 -> out_1/1
  Clock/1 -> Fcn1/1
  Fcn1/1 -> Look-Up Table/1

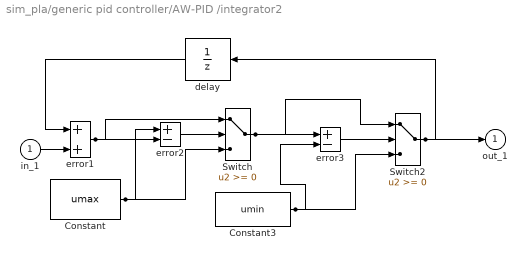
== system sim_pla/generic pid controller/AW-PID /integrator2 ==
  in_1 : Inport  Port=1  PortWidth=-1  SampleTime=-1
  Constant : Constant  Value=umax
  Constant3 : Constant  Value=umin
  Switch : Switch  Threshold=0
  Switch2 : Switch  Threshold=0
  delay : DiscreteTransferFcn  Orientation=left  Numerator=[1]  Denominator=[1 0]  SampleTime=DT
  error1 : Sum  Inputs=++
  error2 : Sum  Inputs=+-
  error3 : Sum  Inputs=+-
  out_1 : Outport  Port=1  InitialOutput=0
  wires:
  delay/1 -> error1/1
  error2/1 -> Switch/2
  error3/1 -> Switch2/2
  Constant3/1 -> error3/2, Switch2/3
  Constant/1 -> error2/1, Switch/3
  error1/1 -> error2/2, Switch/1
  Switch/1 -> error3/1, Switch2/1
  Switch2/1 -> delay/1, out_1/1
  in_1/1 -> error1/2

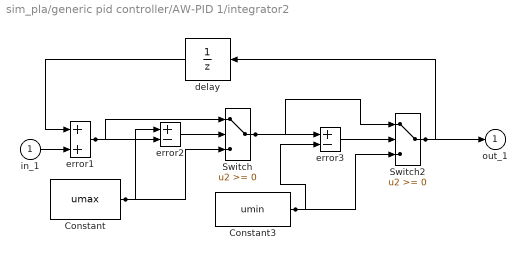
== system sim_pla/generic pid controller/AW-PID 1/integrator2 ==
  in_1 : Inport  Port=1  PortWidth=-1  SampleTime=-1
  Constant : Constant  Value=umax
  Constant3 : Constant  Value=umin
  Switch : Switch  Threshold=0
  Switch2 : Switch  Threshold=0
  delay : DiscreteTransferFcn  Orientation=left  Numerator=[1]  Denominator=[1 0]  SampleTime=DT
  error1 : Sum  Inputs=++
  error2 : Sum  Inputs=+-
  error3 : Sum  Inputs=+-
  out_1 : Outport  Port=1  InitialOutput=0
  wires:
  delay/1 -> error1/1
  error2/1 -> Switch/2
  error3/1 -> Switch2/2
  Constant3/1 -> error3/2, Switch2/3
  Constant/1 -> error2/1, Switch/3
  error1/1 -> error2/2, Switch/1
  Switch/1 -> error3/1, Switch2/1
  Switch2/1 -> delay/1, out_1/1
  in_1/1 -> error1/2

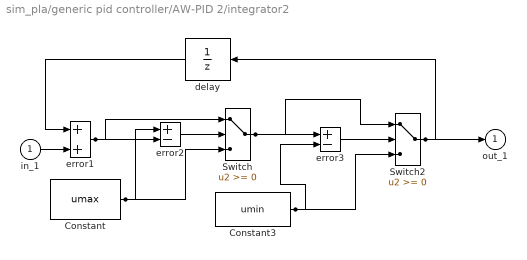
== system sim_pla/generic pid controller/AW-PID 2/integrator2 ==
  in_1 : Inport  Port=1  PortWidth=-1  SampleTime=-1
  Constant : Constant  Value=umax
  Constant3 : Constant  Value=umin
  Switch : Switch  Threshold=0
  Switch2 : Switch  Threshold=0
  delay : DiscreteTransferFcn  Orientation=left  Numerator=[1]  Denominator=[1 0]  SampleTime=DT
  error1 : Sum  Inputs=++
  error2 : Sum  Inputs=+-
  error3 : Sum  Inputs=+-
  out_1 : Outport  Port=1  InitialOutput=0
  wires:
  delay/1 -> error1/1
  error2/1 -> Switch/2
  error3/1 -> Switch2/2
  Constant3/1 -> error3/2, Switch2/3
  Constant/1 -> error2/1, Switch/3
  error1/1 -> error2/2, Switch/1
  Switch/1 -> error3/1, Switch2/1
  Switch2/1 -> delay/1, out_1/1
  in_1/1 -> error1/2
